simulink model "SPGF_FSK_0000_R2020b"  (R2020b)
settings: Solver=ode4  StartTime=0.0  StopTime=1.4  FixedStep=50e-6/50  RelTol=1e-3  EnableMultiTasking=on
undefined symbols (not defined in the file): D11, Delta
libraries: powerlib x2546, powerlib_meascontrol x183, simulink x24
(part 1 of 34)
settings Model: SimulationMode=accelerator  Creator=Anastasia  LastModifiedBy=Fedot
settings DataIOCC: SaveFormat=Array  SaveOutput=off  SignalLogging=off  DSMLogging=off  SaveTime=off  ReturnWorkspaceOutputs=off
settings OptimizationCC: BlockReduction=off  OptimizeBlockIOStorage=off  BufferReuse=off  GlobalBufferReuse=off  ExpressionFolding=off  LocalBlockOutputs=off  EfficientMapNaN2IntZero=off  LifeSpan=inf
settings DebuggingCC: UnderspecifiedInitializationDetection=Classic  MergeDetectMultiDrivingBlocksExec=none  SolverPrmCheckMsg=warning  UnconnectedInputMsg=none  UnconnectedOutputMsg=none  UnconnectedLineMsg=none  AllowSymbolicDim=off  StateNameClashWarn=warning  SFUnexpectedBacktrackingDiag=warning  SFNoUnconditionalDefaultTransitionDiag=warning  SFExecutionAtInitializationDiag=none  ArithmeticOperatorsInVariantConditions=warning
settings HardwareCC: ProdBitPerPointer=32  ProdBitPerSizeT=32  ProdBitPerPtrDiffT=32  ProdLargestAtomicFloat=None  ProdIntDivRoundTo=Undefined  ProdEndianess=Unspecified  ProdWordSize=32  ProdHWDeviceType=32-bit Generic  TargetBitPerPointer=64  TargetBitPerSizeT=64  TargetBitPerPtrDiffT=64  TargetLongLongMode=on  TargetIntDivRoundTo=Zero  TargetEndianess=LittleEndian  TargetWordSize=64  TargetHWDeviceType=MATLAB Host  ProdEqTarget=off
settings ModelReferenceCC: PropagateSignalLabelsOutOfModel=off
settings SFSimCC: SimUseLocalCustomCode=off  CustomCodeUndefinedFunction=UseInterfaceOnly
settings RTWCC: RTWUseLocalCustomCode=off
settings CodeAppCC: MaxIdLength=128  StateflowObjectComments=on
settings GRTTargetCC: TargetLangStandard=C89/C90 (ANSI)  CombineOutputUpdateFcns=off  GRTInterface=on
settings ConfigComp: CovMetricSettings=dw  CovSaveCumulativeToWorkspaceVar=on  CovSaveSingleToWorkspaceVar=on  CovExternalEMLEnable=off
settings SimscapeCC: SimscapeNormalizeSystem=off

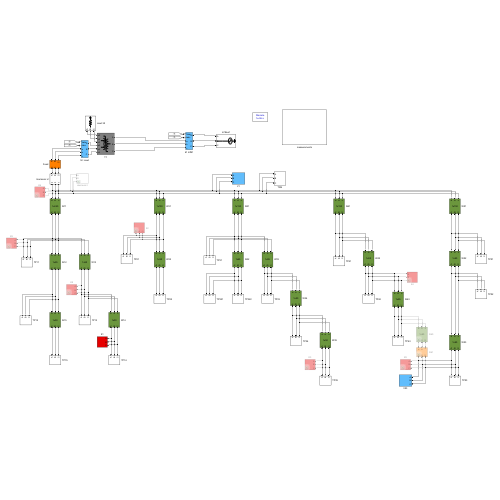
[thumbnail: Simulink's stored preview of the top-level diagram]
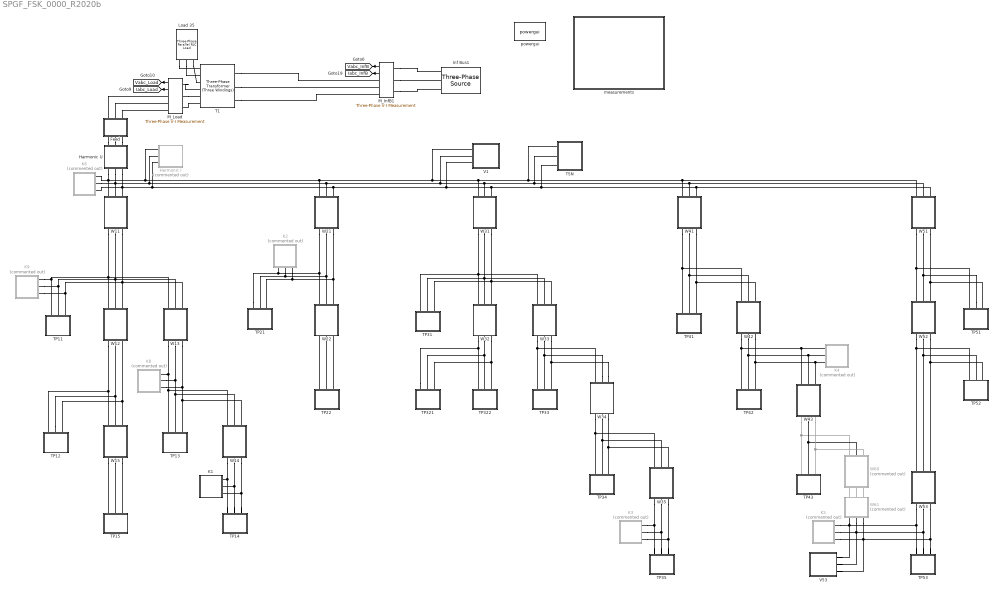
== system SPGF_FSK_0000_R2020b ==
  Feed : Subsystem
      mask Display:
      | port_label('lconn',1,'A');
      | port_label('lconn',2,'B');
      | port_label('lconn',3,'C');
      | 
      | port_label('rconn',1,'a');
      | port_label('rconn',2,'b');
      | port_label('rconn',3,'c');
  Harmonic I : Subsystem  Commented=on  mask(Three-Phase Harmonic Current Source){ActiveABC=[1 0 0], Frequency=50, PhaseABC=[0 -120 120], HN=[5, 7, 11, 13, 17], Current=19.26, Percent=[2.84, 2.42, 1.67, 0.74, 0.3], PhaseH=[0 0 0 0 0]}
      mask prompts: ActiveABC "Active phase of source [A, B, C]"; Frequency "Frequency f [Hz] :"; PhaseABC "Current phase [phA, phB, phC] [degree]"; HN "Vector of harmonic numbers [5, 7, 11, 13 ...] :"; Current "Base current rms [A] :"; Percent "Percent of harmanic in base current [%] :"; PhaseH "Phase of harmonic current [degree] :"
      mask help: Add harmonic to current
      mask init:
      | ActiveA = ActiveABC(1);
      |     ActiveB = ActiveABC(2);
      |     ActiveC = ActiveABC(3);
      |     PhaseA = PhaseABC(1);
      |     PhaseB = PhaseABC(2);
      |     PhaseC = PhaseABC(3);
  Harmonic U : Subsystem  mask(Three-Phase Harmonic Voltage Source){EnableH=off, ActiveABC=[1, 1, 1], Frequency=50, PhaseABC=[0 -120 120], HN=[5, 7, 11, 13, 17], Voltage=1000, Percent=[2.84, 2.42, 1.67, 0.74, 0.3].*1.5, PhaseH=[0 0 0 0 0]}
      mask prompts: EnableH "Enable harmonic voltage source"; ActiveABC "Active phase of source [A, B, C]"; Frequency "Frequency f [Hz] :"; PhaseABC "Voltage phase [phA, phB, phC] [degree]"; HN "Vector of harmonic numbers [5, 7, 11, 13 ...] :"; Voltage "Base Voltage rms [V] :"; Percent "Percent of harmanic in base voltage [%] :"; PhaseH "Phase of harmonic voltage [degree] :"
      mask help:
      | The block allows to add harmonic signals to voltage.
      | The block is connected in series.
      mask init:
      | PhaseA = PhaseABC(1);
      |     PhaseB = PhaseABC(2);
      |     PhaseC = PhaseABC(3);
      |     ActiveA = ActiveABC(1);
      |     ActiveB = ActiveABC(2);
      |     ActiveC = ActiveABC(3);
      mask Callback EnableH:
      | base_block_name = gcb;
      |     enable = get_param(base_block_name, 'EnableH');
      |     if strcmp(enable, 'on')
      |         set_param([base_block_name, '/harmonic'],'Commented','off');
      |         set_param([base_block_name, '/shunt'],'Commented','on');
      |     else
      |         set_param([base_block_name, '/harmonic'],'Commented','on');
      |         set_param([base_block_name, '/shunt'],'Commented','off');
      |     end
  Inf Bus1 : powerlib/Electrical Sources/Three-Phase Source  InternalConnection=Yg  VoltagePhases=off  Voltage=(115500)*1  PhaseAngle=0  Voltage_phases=[25e3 25e3 25e3]/sqrt(3)  PhaseAngles_phases=[0 -120 +120]  Frequency=50  NonIdealSource=on  SpecifyImpedance=off  Resistance=0  Inductance=0  ShortCircuitLevel=100e6  BaseVoltage=115.5e3  XRratio=7  BusType=swing  Pref=0  Qref=0  Prefabc=[10e3, 10e3, 10e3]  Qrefabc=[0, 0, 0]  Qmin=-inf  Qmax=inf
  K1 : Subsystem
  K2 : Subsystem  Commented=on
  K3 : Subsystem  Commented=on
  K4 : Subsystem  Commented=on
  K5 : Subsystem  Commented=on
  K6 : Subsystem  Commented=on
  K8 : Subsystem  Commented=on
  K9 : Subsystem  Commented=on
  Load 35 : powerlib/Elements/Three-Phase Parallel RLC Load  LConnTagsString=A|B|C  Configuration=Y (grounded)  NominalVoltage=(38435.4)*1  Vabc=[1e3 1e3 1e3]  Vabcp=[1e3 1e3 1e3]  NominalFrequency=50  UnbalancedPower=off  ActivePower=1e6  InductivePower=0  CapacitivePower=0  Pabc=[10e3 9e3 11e3]  QLabc=[100 90 110]  QCabc=[100 90 110]  Pabcp=[10e3 9e3 11e3]  QLabcp=[100 90 110]  QCabcp=[100 90 110]  Measurements=None  LoadType=constant PQ
  M_InfB1 : powerlib/Measurements/Three-Phase V-I Measurement  VoltageMeasurement=phase-to-ground  SetLabelV=off  LabelV=Vabc  Vpu=off  VpuLL=off  CurrentMeasurement=yes  SetLabelI=off  LabelI=Iabc  Ipu=off  Pbase=100e6  Vbase=500e3  OutputType=Complex  PhasorSimulation=off  PSBequivalent=0
  M_Load : powerlib/Measurements/Three-Phase V-I Measurement  VoltageMeasurement=phase-to-ground  SetLabelV=off  LabelV=Vabc  Vpu=off  VpuLL=off  CurrentMeasurement=yes  SetLabelI=off  LabelI=Iabc  Ipu=off  Pbase=100e6  Vbase=500e3  OutputType=Complex  PhasorSimulation=off  PSBequivalent=0
  T1 : powerlib/Elements/Three-Phase Transformer (Three Windings)  Winding1Connection=Yg  Winding2Connection=Y  Winding3Connection=Delta (D11)  CoreType=Three single-phase transformers  SetSaturation=on  Hysteresis=off  DataFile='hysteresis'  SetInitialFlux=off  Measurements=None  UNITS=pu  NominalPower=[20e6 , 50 ]  Winding1=[115.5e3 , 0.003175 , 0.01025 ]  Winding2=[ 38.5e3 , 0.003175 , -0.0025]  Winding3="[ 11e3 , 0.003175 ,  0.0125 ]"  Rm=444.444  Lm=40  L0=2  Saturation=[0 0;0.01774 0.324129;0.0487637 0.61284;0.0980856 0.825118;0.2 1;0.309543 1.08024;0.652348 1.17344;2.0357 1.26115;6.0215 1.36094;12.4388 1.49469]  InitialFluxes=[-0.996027177222096 0.502063669050077 0.493963508171988]  BreakLoop=on  DiscreteSolver=Trapezoidal iterative  DataType=off  TransfoNumber=1
  TP11 : Subsystem
  TP12 : Subsystem
  TP13 : Subsystem
  TP14 : Subsystem
  TP15 : Subsystem
  TP21 : Subsystem
  TP22 : Subsystem
  TP31 : Subsystem
  TP321 : Subsystem
  TP322 : Subsystem
  TP33 : Subsystem
  TP34 : Subsystem
  TP35 : Subsystem
  TP41 : Subsystem
  TP42 : Subsystem
  TP43 : Subsystem
  TP51 : Subsystem
  TP52 : Subsystem
  TP53 : Subsystem
  TSN : Subsystem
  V1 : Subsystem
  V53 : Subsystem
  W11 : Subsystem
      mask Display:
      | port_label('lconn',1,'A');
      | port_label('lconn',2,'B');
      | port_label('lconn',3,'C');
      | 
      | port_label('rconn',1,'a');
      | port_label('rconn',2,'b');
      | port_label('rconn',3,'c');
      | disp('1x240');
  W12 : Subsystem
      mask Display:
      | port_label('lconn',1,'A');
      | port_label('lconn',2,'B');
      | port_label('lconn',3,'C');
      | 
      | port_label('rconn',1,'a');
      | port_label('rconn',2,'b');
      | port_label('rconn',3,'c');
      | disp('1x95');
  W13 : Subsystem
      mask Display:
      | port_label('lconn',1,'A');
      | port_label('lconn',2,'B');
      | port_label('lconn',3,'C');
      | 
      | port_label('rconn',1,'a');
      | port_label('rconn',2,'b');
      | port_label('rconn',3,'c');
      | disp('1x95');
  W14 : Subsystem
      mask Display:
      | port_label('lconn',1,'A');
      | port_label('lconn',2,'B');
      | port_label('lconn',3,'C');
      | 
      | port_label('rconn',1,'a');
      | port_label('rconn',2,'b');
      | port_label('rconn',3,'c');
      | disp('1x50');
  W15 : Subsystem
      mask Display:
      | port_label('lconn',1,'A');
      | port_label('lconn',2,'B');
      | port_label('lconn',3,'C');
      | 
      | port_label('rconn',1,'a');
      | port_label('rconn',2,'b');
      | port_label('rconn',3,'c');
      | disp('1x50');
  W21 : Subsystem
      mask Display:
      | port_label('lconn',1,'A');
      | port_label('lconn',2,'B');
      | port_label('lconn',3,'C');
      | 
      | port_label('rconn',1,'a');
      | port_label('rconn',2,'b');
      | port_label('rconn',3,'c');
      | disp('1x150');
  W22 : Subsystem
      mask Display:
      | port_label('lconn',1,'A');
      | port_label('lconn',2,'B');
      | port_label('lconn',3,'C');
      | 
      | port_label('rconn',1,'a');
      | port_label('rconn',2,'b');
      | port_label('rconn',3,'c');
      | disp('1x95');
  W31 : Subsystem
      mask Display:
      | port_label('lconn',1,'A');
      | port_label('lconn',2,'B');
      | port_label('lconn',3,'C');
      | 
      | port_label('rconn',1,'a');
      | port_label('rconn',2,'b');
      | port_label('rconn',3,'c');
      | disp('1x150');
  W32 : Subsystem
      mask Display:
      | port_label('lconn',1,'A');
      | port_label('lconn',2,'B');
      | port_label('lconn',3,'C');
      | 
      | port_label('rconn',1,'a');
      | port_label('rconn',2,'b');
      | port_label('rconn',3,'c');
      | disp('1x95');
  W33 : Subsystem
      mask Display:
      | port_label('lconn',1,'A');
      | port_label('lconn',2,'B');
      | port_label('lconn',3,'C');
      | 
      | port_label('rconn',1,'a');
      | port_label('rconn',2,'b');
      | port_label('rconn',3,'c');
      | disp('1x95');
  W34 : Subsystem
      mask Display:
      | port_label('lconn',1,'A');
      | port_label('lconn',2,'B');
      | port_label('lconn',3,'C');
      | 
      | port_label('rconn',1,'a');
      | port_label('rconn',2,'b');
      | port_label('rconn',3,'c');
      | disp('1x50');
  W35 : Subsystem
      mask Display:
      | port_label('lconn',1,'A');
      | port_label('lconn',2,'B');
      | port_label('lconn',3,'C');
      | 
      | port_label('rconn',1,'a');
      | port_label('rconn',2,'b');
      | port_label('rconn',3,'c');
      | disp('1x50');
  W41 : Subsystem
      mask Display:
      | port_label('lconn',1,'A');
      | port_label('lconn',2,'B');
      | port_label('lconn',3,'C');
      | 
      | port_label('rconn',1,'a');
      | port_label('rconn',2,'b');
      | port_label('rconn',3,'c');
      | disp('1x150');
  W42 : Subsystem
      mask Display:
      | port_label('lconn',1,'A');
      | port_label('lconn',2,'B');
      | port_label('lconn',3,'C');
      | 
      | port_label('rconn',1,'a');
      | port_label('rconn',2,'b');
      | port_label('rconn',3,'c');
      | disp('1x95');
  W43 : Subsystem
      mask Display:
      | port_label('lconn',1,'A');
      | port_label('lconn',2,'B');
      | port_label('lconn',3,'C');
      | 
      | port_label('rconn',1,'a');
      | port_label('rconn',2,'b');
      | port_label('rconn',3,'c');
      | disp('1x95');
  W51 : Subsystem
      mask Display:
      | port_label('lconn',1,'A');
      | port_label('lconn',2,'B');
      | port_label('lconn',3,'C');
      | 
      | port_label('rconn',1,'a');
      | port_label('rconn',2,'b');
      | port_label('rconn',3,'c');
      | disp('1x150');
  W52 : Subsystem
      mask Display:
      | port_label('lconn',1,'A');
      | port_label('lconn',2,'B');
      | port_label('lconn',3,'C');
      | 
      | port_label('rconn',1,'a');
      | port_label('rconn',2,'b');
      | port_label('rconn',3,'c');
      | disp('1x95');
  W53 : Subsystem
      mask Display:
      | port_label('lconn',1,'A');
      | port_label('lconn',2,'B');
      | port_label('lconn',3,'C');
      | 
      | port_label('rconn',1,'a');
      | port_label('rconn',2,'b');
      | port_label('rconn',3,'c');
      | disp('1x95');
  W60 : Subsystem  Commented=on
      mask Display:
      | port_label('lconn',1,'A');
      | port_label('lconn',2,'B');
      | port_label('lconn',3,'C');
      | 
      | port_label('rconn',1,'a');
      | port_label('rconn',2,'b');
      | port_label('rconn',3,'c');
      | disp('1x95');
  W61 : Subsystem  Commented=on
      mask Display:
      | port_label('lconn',1,'A');
      | port_label('lconn',2,'B');
      | port_label('lconn',3,'C');
      | 
      | port_label('rconn',1,'a');
      | port_label('rconn',2,'b');
      | port_label('rconn',3,'c');
  measurements : Subsystem  mask{FTime=0.02/40}
      mask prompts: FTime "Fourier Sample Time"
  powergui : powerlib/powergui  Priority=1  SimulationMode=Discrete  SampleTime=50e-6/50  frequency=60  Iterations=100  frequencyindice=0  Pbase=1e+06  ErrMax=0.0001  UnitsV=kV  UnitsW=MW  buscounter=0  FunctionMessages=off  echomessages=off  EnableUseOfTLC=off  CurrentSourceSwitches=off  DisableSnubberDevices=off  DisableRonSwitches=off  DisableVfSwitches=off  DisplayEquations=off  AutomaticDiscreteSolvers=off  SolverType=Backward Euler  Interpol=off  ExternalGateDelay=off  methode=off  Ts=0  x0status=blocks  SPID=off  SwTol=0  HookPort=off  NonlinearTolerance=1e-4  nMaxIteration=100  ContinueOnMaxIteration=off  RestoreLinks=warning  ResistiveCurrentMeasurement=off  Frange=[0:2:500]  Ylog=off  Xlog=on  ShowGrid=off  save=off  variable=ZData  structure=0  ZoomFFT=off  StartTime=0.0  cycles=1  DisplayStyle=1  fundamental=60  FreqAxis=off  MaxFrequency=1000  frequencyindicesteady=1  RmsSteady=2  display=off
  tag scope: Iabc_InfB=global, Iabc_Load=global, Vabc_InfB=global, Vabc_Load=global
  wires:
  M_InfB1/1 -> [Vabc_InfB]
  M_InfB1/2 -> [Iabc_InfB]
  M_Load/1 -> [Vabc_Load]
  M_Load/2 -> [Iabc_Load]
  connections:
  M_InfB1/LConn1 -- Inf Bus1/RConn1
  TP12/RConn2 -- W15/RConn2 -- W12/LConn2
  W12/LConn3 -- W15/RConn3 -- TP12/RConn3
  W15/RConn1 -- TP12/RConn1 -- W12/LConn1
  W13/LConn1 -- K8/LConn1 -- W14/RConn1 -- TP13/RConn1
  W13/LConn2 -- K8/LConn2 -- W14/RConn2 -- TP13/RConn2
  W14/RConn3 -- K8/LConn3 -- W13/LConn3 -- TP13/RConn3
  W14/LConn1 -- TP14/RConn1 -- K1/LConn1
  K1/LConn2 -- TP14/RConn2 -- W14/LConn2
  TP21/RConn1 -- K2/LConn1 -- W22/RConn1 -- W21/LConn1
  TP21/RConn3 -- K2/LConn3 -- W22/RConn3 -- W21/LConn3
  TP21/RConn2 -- K2/LConn2 -- W22/RConn2 -- W21/LConn2
  W33/RConn2 -- TP31/RConn2 -- W32/RConn2 -- W31/LConn2
  W33/RConn3 -- TP31/RConn3 -- W32/RConn3 -- W31/LConn3
  W33/RConn1 -- TP31/RConn1 -- W32/RConn1 -- W31/LConn1
  TP321/RConn1 -- TP322/RConn1 -- W32/LConn1
  TP321/RConn2 -- TP322/RConn2 -- W32/LConn2
  TP322/RConn3 -- TP321/RConn3 -- W32/LConn3
  W34/RConn3 -- TP33/RConn3 -- W33/LConn3
  W34/RConn1 -- TP33/RConn1 -- W33/LConn1
  W34/RConn2 -- TP33/RConn2 -- W33/LConn2
  W35/RConn3 -- TP34/RConn3 -- W34/LConn3
  W35/RConn1 -- TP34/RConn1 -- W34/LConn1
  W35/RConn2 -- TP34/RConn2 -- W34/LConn2
  TP35/RConn3 -- K3/LConn3 -- W35/LConn3
  TP35/RConn1 -- K3/LConn1 -- W35/LConn1
  TP35/RConn2 -- K3/LConn2 -- W35/LConn2
  W42/RConn2 -- TP41/RConn2 -- W41/LConn2
  W42/RConn1 -- TP41/RConn1 -- W41/LConn1
  W42/RConn3 -- TP41/RConn3 -- W41/LConn3
  W43/RConn3 -- K4/LConn3 -- TP42/RConn3 -- W42/LConn3
  W43/RConn1 -- K4/LConn1 -- TP42/RConn1 -- W42/LConn1
  TP42/RConn2 -- W42/LConn2 -- K4/LConn2 -- W43/RConn2
  W60/RConn1 -- TP43/RConn1 -- W43/LConn1
  TP43/RConn2 -- W60/RConn2 -- W43/LConn2
  W60/RConn3 -- TP43/RConn3 -- W43/LConn3
  W51/LConn3 -- TP51/RConn3 -- W52/RConn3
  W52/RConn1 -- TP51/RConn1 -- W51/LConn1
  TP51/RConn2 -- W51/LConn2 -- W52/RConn2
  TP52/RConn2 -- W53/RConn2 -- W52/LConn2
  TP52/RConn3 -- W53/RConn3 -- W52/LConn3
  TP52/RConn1 -- W53/RConn1 -- W52/LConn1
  T1/LConn2 -- M_InfB1/RConn2
  M_InfB1/LConn2 -- Inf Bus1/RConn2
  Load 35/LConn2 -- T1/RConn2
  M_InfB1/LConn3 -- Inf Bus1/RConn3
  T1/LConn3 -- M_InfB1/RConn3
  T1/LConn1 -- M_InfB1/RConn1
  Load 35/LConn1 -- T1/RConn1
  Load 35/LConn3 -- T1/RConn3
  W15/LConn1 -- TP15/RConn1
  W15/LConn2 -- TP15/RConn2
  TP22/RConn3 -- W22/LConn3
  TP22/RConn1 -- W22/LConn1
  TP22/RConn2 -- W22/LConn2
  W15/LConn3 -- TP15/RConn3
  M_Load/LConn3 -- T1/RConn6
  M_Load/LConn2 -- T1/RConn5
  M_Load/LConn1 -- T1/RConn4
  Feed/LConn1 -- M_Load/RConn1
  Feed/LConn2 -- M_Load/RConn2
  Feed/LConn3 -- M_Load/RConn3
  W14/LConn3 -- TP14/RConn3 -- K1/LConn3
  W11/LConn3 -- K9/LConn3 -- TP11/RConn3 -- W13/RConn3 -- W12/RConn3
  W11/LConn1 -- K9/LConn1 -- TP11/RConn1 -- W13/RConn1 -- W12/RConn1
  W61/LConn2 -- K5/LConn2 -- V53/LConn2 -- TP53/RConn2 -- W53/LConn2
  W61/LConn1 -- K5/LConn1 -- V53/LConn1 -- TP53/RConn1 -- W53/LConn1
  W61/LConn3 -- K5/LConn3 -- V53/LConn3 -- TP53/RConn3 -- W53/LConn3
  Harmonic U/RConn1 -- K6/LConn1 -- W11/RConn1 -- Harmonic I/LConn1 -- W21/RConn1 -- V1/LConn1 -- W31/RConn1 -- TSN/LConn1 -- W51/RConn1 -- W41/RConn1
  Harmonic I/LConn2 -- Harmonic U/RConn2 -- K6/LConn2 -- W11/RConn2 -- W21/RConn2 -- V1/LConn2 -- W51/RConn2 -- W41/RConn2 -- TSN/LConn2 -- W31/RConn2
  TSN/LConn3 -- Harmonic I/LConn3 -- Harmonic U/RConn3 -- W11/RConn3 -- K6/LConn3 -- W21/RConn3 -- V1/LConn3 -- W31/RConn3 -- W51/RConn3 -- W41/RConn3
  W61/RConn1 -- W60/LConn1
  W61/RConn2 -- W60/LConn2
  W61/RConn3 -- W60/LConn3
  TP11/RConn2 -- K9/LConn2 -- W11/LConn2 -- W12/RConn2 -- W13/RConn2
  Feed/RConn1 -- Harmonic U/LConn1
  Feed/RConn2 -- Harmonic U/LConn2
  Feed/RConn3 -- Harmonic U/LConn3

== system SPGF_FSK_0000_R2020b/Feed ==
  Q : Subsystem
  A : PMIOPort  Side=Left
  B : PMIOPort  Port=2  Side=Left
  C : PMIOPort  Port=3  Side=Left
  a : PMIOPort  Port=4  Side=Right
  b : PMIOPort  Port=5  Side=Right
  c : PMIOPort  Port=6  Side=Right
  connections:
  Q/RConn3 -- C/RConn1
  Q/RConn2 -- B/RConn1
  Q/LConn2 -- b/RConn1
  Q/LConn1 -- a/RConn1
  Q/LConn3 -- c/RConn1
  Q/RConn1 -- A/RConn1

== system SPGF_FSK_0000_R2020b/Harmonic I ==
  Clock : Clock
  Constant1 : Constant  Value=PhaseB
  Constant2 : Constant  Value=PhaseC
  Constant3 : Constant  Value=PhaseA
  Constant4 : Constant  Value=ActiveA
  Constant5 : Constant  Value=ActiveB
  Constant6 : Constant  Value=ActiveC
  Ground : powerlib/Elements/Ground  LConnTagsString=a
  In A : powerlib/Electrical Sources/Controlled Current Source  Initialize=on  Source_Type=AC  Amplitude=0  Phase=0  Frequency=50  Measurements=None
  In B : powerlib/Electrical Sources/Controlled Current Source  Initialize=on  Source_Type=AC  Amplitude=0  Phase=-120  Frequency=50  Measurements=None
  In C : powerlib/Electrical Sources/Controlled Current Source  Initialize=on  Source_Type=AC  Amplitude=0  Phase=120  Frequency=50  Measurements=None
  Product1 : Product
  Product15 : Product
  Product2 : Product
  R : powerlib/Elements/Three-Phase Series RLC Branch  LConnTagsString=A|B|C  RConnTagsString=A|B|C  BranchType=R  Resistance=1e6  Inductance=0  Capacitance=0  Measurements=None
  Subsystem1 : Subsystem
  Subsystem2 : Subsystem
  Subsystem3 : Subsystem
  Sum of Elements : Sum  Inputs=+
  Sum of Elements1 : Sum  Inputs=+
  Sum of Elements2 : Sum  Inputs=+
  A : PMIOPort  Tag=PMCPort  Side=Left
  B : PMIOPort  Tag=PMCPort  Port=2  Side=Left
  C : PMIOPort  Tag=PMCPort  Port=3  Side=Left
  wires:
  Product2/1 -> In C/1
  Constant6/1 -> Product2/1
  Product1/1 -> In B/1
  Constant5/1 -> Product1/1
  Product15/1 -> In A/1
  Constant4/1 -> Product15/1
  Subsystem3/1(o) -> Sum of Elements/1
  Subsystem1/1(o) -> Sum of Elements1/1
  Subsystem2/1(o) -> Sum of Elements2/1
  Sum of Elements/1 -> Product15/2
  Sum of Elements1/1 -> Product1/2
  Sum of Elements2/1 -> Product2/2
  Constant3/1 -> Subsystem3/2(phase)
  Constant1/1 -> Subsystem1/2(phase)
  Clock/1 -> Subsystem3/1(clock), Subsystem2/1(clock), Subsystem1/1(clock)
  Constant2/1 -> Subsystem2/2(phase)
  connections:
  R/RConn1 -- In A/RConn1
  In B/RConn1 -- R/RConn2
  R/RConn3 -- In C/RConn1
  In C/LConn1 -- Ground/LConn1 -- In A/LConn1 -- In B/LConn1
  B/RConn1 -- R/LConn2
  C/RConn1 -- R/LConn3
  A/RConn1 -- R/LConn1

== system SPGF_FSK_0000_R2020b/Harmonic U ==
  harmonic : Subsystem  Commented=on
  shunt : Subsystem
  A : PMIOPort  Tag=PMCPort  Side=Left
  B : PMIOPort  Tag=PMCPort  Port=2  Side=Left
  C : PMIOPort  Tag=PMCPort  Port=3  Side=Left
  a : PMIOPort  Port=4  Side=Right
  b : PMIOPort  Port=5  Side=Right
  c : PMIOPort  Port=6  Side=Right
  connections:
  harmonic/LConn1 -- shunt/LConn3 -- A/RConn1
  harmonic/RConn3 -- shunt/RConn3 -- c/RConn1
  b/RConn1 -- harmonic/RConn2 -- shunt/RConn2
  a/RConn1 -- harmonic/RConn1 -- shunt/RConn1
  harmonic/LConn3 -- shunt/LConn2 -- C/RConn1
  harmonic/LConn2 -- shunt/LConn1 -- B/RConn1

== system SPGF_FSK_0000_R2020b/K1 ==
  fault : Subsystem  mask{FaultA=on, FaultB=off, FaultC=off, FaultResistance=0.0001, GroundResistance=1e-03, SnubberResistance=1e6, SnubberCapacitance=inf, TransitionTimes=[0.2 0.8], TheoryOfArc=Peters & Slepian, ArcingVoltage=6000, TypeOfPause=None, NoiseSampleTime=0.04, NoiseSeed=23345, PulsePeriod=0.2, PulseWidth=20, PhaseDelay=0.2, SwitchTimes=[0.2 0.225 0.5 0.6], LimitArcNum=off, ArcingNumber=2, AddTimeDelay=off, TimeDelay=[0 0.1 0.2 ]}
      mask prompts: FaultA "Phase A Fault"; FaultB "Phase B Fault"; FaultC "Phase C Fault"; FaultResistance "Fault resistance Ron (ohms) :"; GroundResistance "Ground resistance Rg (ohms) :"; SnubberResistance "Snubbers resistance Rp (ohms) :"; SnubberCapacitance "Snubbers capacitance Cp (F) :"; TransitionTimes "Transition times (s) :"; TheoryOfArc "Theory of the arcing ground"; ArcingVoltage "Voltage of the arcing (V) :"; TypeOfPause "Add pause in the arcing ground"; NoiseSampleTime "Sample time of white noise (s) :"; NoiseSeed "Seed of white noise"; PulsePeriod "Period of pulses (s) :"; PulseWidth "Width of pulse (% of period) :"; PhaseDelay "Phase delay (sec) :"; SwitchTimes "Switch times (sec) [1,0,1,0...] :"; LimitArcNum "Limit number of arcing [N] :"; ArcingNumber "Number of uprising arcing"; AddTimeDelay "Add time delay :"; TimeDelay "Time delay between arc (sec) [1xN] :"
      mask init:
      | FaultA = double(FaultA);
      | FaultB = double(FaultB);
      | FaultC = double(FaultC);
      | if (FaultA == 1)
      |     FaultPhase = 1;
      | elseif (FaultB == 1)
      |     FaultPhase = 2;    
      | elseif (FaultC == 1)
      |     FaultPhase = 3; 
      | else
      |     FaultPhase = 4; 
      | end
      |     BeginFaultTime = TransitionTimes(1);
      |     EndFaultTime = TransitionTimes(2);
      | if (length(ArcingVoltage) == 1)
      |     Slope = 0;
      | end
      | if (length(ArcingVoltage) > 1)
      |     Slope = (ArcingVoltage(2)-ArcingVoltage(1))/(EndFaultTime-BeginFaultTime);
      | end
      | 
      | SwitchStatus(1) = 0;
      | for i=1:length(SwitchTimes)
      |     SwitchStatus(i+1) = double(~(logical(SwitchStatus(i))));
      | end
      | SwitchTimes = [0,SwitchTimes];
      | 
      | LimitArcNum = double(LimitArcNum);
      | AddTimeDelay = double(AddTimeDelay);
      | 
      | if (AddTimeDelay == 0)
      |     TimeDelay = zeros(1,ArcingNumber);
      | end
      settings: CloseFcn=|
      | en = get_param(gcb,'MaskEnables');
      | set_param(gcb,'MaskEnables',en)
      | clear enab en;
      settings: MoveFcn=|
      | en = get_param(gcb,'MaskEnables');
      | set_param(gcb,'MaskEnables',en)
      | clear enab en;
      mask Callback FaultA:
      | enab = get_param(gcb,'FaultA');
      | en = get_param(gcb,'MaskEnables');
      | % Set the 'MaskVisililities' property for each parameters
      | if strcmp(enab,'on')
      |     en{2}='off';
      |     en{3}='off';
      | % set_param(gcb,'MaskVisibilities',{'on','on','on','on','on','on','on','on','on','off','on','',''});
      | else
      |     en{2}='on';
      |     en{3}='on';
      | % set_param(gcb,'MaskVisibilities',{'on','on','on','on','on','on','on','on','on','on','on','',''});
      | end
      | set_param(gcb,'MaskEnables',en)
      | clear enab en;
      mask Callback FaultB:
      | enab = get_param(gcb,'FaultB');
      | en = get_param(gcb,'MaskEnables');
      | % Set the 'MaskVisililities' property for each parameters
      | if strcmp(enab,'on')
      |     en{1}='off';
      |     en{3}='off';
      | % set_param(gcb,'MaskVisibilities',{'on','on','on','on','on','on','on','on','on','off','on','',''});
      | else
      |     en{1}='on';
      |     en{3}='on';
      | % set_param(gcb,'MaskVisibilities',{'on','on','on','on','on','on','on','on','on','on','on','',''});
      | end
      | set_param(gcb,'MaskEnables',en)
      | clear enab en;
      mask Callback FaultC:
      | enab = get_param(gcb,'FaultC');
      | en = get_param(gcb,'MaskEnables');
      | % Set the 'MaskVisililities' property for each parameters
      | if strcmp(enab,'on')
      |     en{1}='off';
      |     en{2}='off';
      | % set_param(gcb,'MaskVisibilities',{'on','on','on','on','on','on','on','on','on','off','on','',''});
      | else
      |     en{1}='on';
      |     en{2}='on';
      | % set_param(gcb,'MaskVisibilities',{'on','on','on','on','on','on','on','on','on','on','on','',''});
      | end
      | set_param(gcb,'MaskEnables',en)
      | clear enab en;
      mask TypeOptions TheoryOfArc: None | Petersen | Peters & Slepian
      mask Callback TheoryOfArc:
      | enab = get_param(gcb,'TheoryOfArc');
      | en = get_param(gcb,'MaskEnables');
      | % Set the 'MaskVisililities' property for each parameters
      | if strcmp(enab,'None')
      |     en{10}='off';
      | % set_param(gcb,'MaskVisibilities',{'on','on','on','on','on','on','on','on','on','off','on','',''});
      | else
      |     en{10}='on';
      | % set_param(gcb,'MaskVisibilities',{'on','on','on','on','on','on','on','on','on','on','on','',''});
      | end
      | set_param(gcb,'MaskEnables',en)
      | clear enab en;
      mask TypeOptions TypeOfPause: None | White Noise | Pulse Generator | Time Dependent Pulses
      mask Callback TypeOfPause:
      | enab = get_param(gcb,'TypeOfPause');
      | en = get_param(gcb,'MaskVisibilities');
      | % Set the 'MaskVisibilities' property for each parameters
      | if strcmp(enab,'None')
      |     en{12} = 'off';
      |     en{13} = 'off';
      |     en{14} = 'off';
      |     en{15} = 'off';
      |     en{16} = 'off';
      |     en{17} = 'off';
      | % set_param(gcb,'MaskEnables',{'on','on','on','on','on','on','on','on','on','on','on','on','on'});
      | elseif strcmp(enab,'White Noise')
      |     en{12} = 'on';
      |     en{13} = 'on';
      |     en{14} = 'off';
      |     en{15} = 'off';
      |     en{16} = 'off';
      |     en{17} = 'off';
      | elseif strcmp(enab,'Pulse Generator')
      |     en{12} = 'off';
      |     en{13} = 'off';
      |     en{14} = 'on';
      |     en{15} = 'on';
      |     en{16} = 'on';
      |     en{17} = 'off';
      | else
      |     en{12} = 'off';
      |     en{13} = 'off';
      |     en{14} = 'off';
      |     en{15} = 'off';
      |     en{16} = 'off';
      |     en{17} = 'on';
      | % set_param(gcb,'Maskenables',{'on','on','on','on','on','on','on','on','on','on','on','off','off'});
      | end
      | set_param(gcb,'MaskVisibilities',en);
      | clear enab en;
      mask Callback LimitArcNum:
      | enab = get_param(gcb,'LimitArcNum');
      | en = get_param(gcb,'MaskVisibilities');
      | % Set the 'MaskVisibilities' property for each parameters
      | if strcmp(enab,'on')
      |     en{19} = 'on';
      |     en{20} = 'on';
      |     en{21} = 'on';
      | else
      |     en{19} = 'off';
      |     en{20} = 'off';
      |     set_param(gcb,'AddTimeDelay','off');
      |     en{21} = 'off';
      | % set_param(gcb,'Maskenables',{'on','on','on','on','on','on','on','on','on','on','on','off','off'});
      | end
      | set_param(gcb,'MaskVisibilities',en);
      | clear enab en;
      mask Callback AddTimeDelay:
      | enab = get_param(gcb,'AddTimeDelay');
      | en = get_param(gcb,'MaskVisibilities');
      | % Set the 'MaskVisibilities' property for each parameters
      | if strcmp(enab,'on')
      |     en{21} = 'on';
      | else
      |     en{21} = 'off';
      | % set_param(gcb,'Maskenables',{'on','on','on','on','on','on','on','on','on','on','on','off','off'});
      | end
      | set_param(gcb,'MaskVisibilities',en);
      | clear enab en;
      mask Display:
      | % port_label('input',1,'Iabc');
      | 
      | port_label('lconn',1,'A');
      | port_label('lconn',2,'B');
      | port_label('lconn',3,'C');
      | 
      | disp('   ПДЗ    ');
  meas : Subsystem
  A : PMIOPort  Side=Left
  B : PMIOPort  Port=2  Side=Left
  C : PMIOPort  Port=3  Side=Left
  connections:
  meas/LConn3 -- C/RConn1
  meas/LConn1 -- A/RConn1
  meas/LConn2 -- B/RConn1
  fault/LConn3 -- meas/RConn3
  fault/LConn2 -- meas/RConn2
  fault/LConn1 -- meas/RConn1

== system SPGF_FSK_0000_R2020b/K2 ==
  fault : Subsystem  mask{FaultA=on, FaultB=off, FaultC=off, FaultResistance=0.0001, GroundResistance=1e-03, SnubberResistance=1e6, SnubberCapacitance=inf, TransitionTimes=[0.2 0.8], TheoryOfArc=None, ArcingVoltage=6000, TypeOfPause=None, NoiseSampleTime=0.04, NoiseSeed=23345, PulsePeriod=0.2, PulseWidth=20, PhaseDelay=0, SwitchTimes=[0.2 0.225 0.5 0.6], LimitArcNum=off, ArcingNumber=1, AddTimeDelay=off, TimeDelay=[0 0.1 0.2 ]}
      mask prompts: FaultA "Phase A Fault"; FaultB "Phase B Fault"; FaultC "Phase C Fault"; FaultResistance "Fault resistance Ron (ohms) :"; GroundResistance "Ground resistance Rg (ohms) :"; SnubberResistance "Snubbers resistance Rp (ohms) :"; SnubberCapacitance "Snubbers capacitance Cp (F) :"; TransitionTimes "Transition times (s) :"; TheoryOfArc "Theory of the arcing ground"; ArcingVoltage "Voltage of the arcing (V) :"; TypeOfPause "Add pause in the arcing ground"; NoiseSampleTime "Sample time of white noise (s) :"; NoiseSeed "Seed of white noise"; PulsePeriod "Period of pulses (s) :"; PulseWidth "Width of pulse (% of period) :"; PhaseDelay "Phase delay (sec) :"; SwitchTimes "Switch times (sec) [1,0,1,0...] :"; LimitArcNum "Limit number of arcing [N] :"; ArcingNumber "Number of uprising arcing"; AddTimeDelay "Add time delay :"; TimeDelay "Time delay between arc (sec) [1xN] :"
      mask init: same as SPGF_FSK_0000_R2020b/K1/fault
      settings: CloseFcn=|
      | en = get_param(gcb,'MaskEnables');
      | set_param(gcb,'MaskEnables',en)
      | clear enab en;
      settings: MoveFcn=|
      | en = get_param(gcb,'MaskEnables');
      | set_param(gcb,'MaskEnables',en)
      | clear enab en;
      mask Callback FaultA:
      | enab = get_param(gcb,'FaultA');
      | en = get_param(gcb,'MaskEnables');
      | % Set the 'MaskVisililities' property for each parameters
      | if strcmp(enab,'on')
      |     en{2}='off';
      |     en{3}='off';
      | % set_param(gcb,'MaskVisibilities',{'on','on','on','on','on','on','on','on','on','off','on','',''});
      | else
      |     en{2}='on';
      |     en{3}='on';
      | % set_param(gcb,'MaskVisibilities',{'on','on','on','on','on','on','on','on','on','on','on','',''});
      | end
      | set_param(gcb,'MaskEnables',en)
      | clear enab en;
      mask Callback FaultB:
      | enab = get_param(gcb,'FaultB');
      | en = get_param(gcb,'MaskEnables');
      | % Set the 'MaskVisililities' property for each parameters
      | if strcmp(enab,'on')
      |     en{1}='off';
      |     en{3}='off';
      | % set_param(gcb,'MaskVisibilities',{'on','on','on','on','on','on','on','on','on','off','on','',''});
      | else
      |     en{1}='on';
      |     en{3}='on';
      | % set_param(gcb,'MaskVisibilities',{'on','on','on','on','on','on','on','on','on','on','on','',''});
      | end
      | set_param(gcb,'MaskEnables',en)
      | clear enab en;
      mask Callback FaultC:
      | enab = get_param(gcb,'FaultC');
      | en = get_param(gcb,'MaskEnables');
      | % Set the 'MaskVisililities' property for each parameters
      | if strcmp(enab,'on')
      |     en{1}='off';
      |     en{2}='off';
      | % set_param(gcb,'MaskVisibilities',{'on','on','on','on','on','on','on','on','on','off','on','',''});
      | else
      |     en{1}='on';
      |     en{2}='on';
      | % set_param(gcb,'MaskVisibilities',{'on','on','on','on','on','on','on','on','on','on','on','',''});
      | end
      | set_param(gcb,'MaskEnables',en)
      | clear enab en;
      mask TypeOptions TheoryOfArc: None | Petersen | Peters & Slepian
      mask Callback TheoryOfArc:
      | enab = get_param(gcb,'TheoryOfArc');
      | en = get_param(gcb,'MaskEnables');
      | % Set the 'MaskVisililities' property for each parameters
      | if strcmp(enab,'None')
      |     en{10}='off';
      | % set_param(gcb,'MaskVisibilities',{'on','on','on','on','on','on','on','on','on','off','on','',''});
      | else
      |     en{10}='on';
      | % set_param(gcb,'MaskVisibilities',{'on','on','on','on','on','on','on','on','on','on','on','',''});
      | end
      | set_param(gcb,'MaskEnables',en)
      | clear enab en;
      mask TypeOptions TypeOfPause: None | White Noise | Pulse Generator | Time Dependent Pulses
      mask Callback TypeOfPause:
      | enab = get_param(gcb,'TypeOfPause');
      | en = get_param(gcb,'MaskVisibilities');
      | % Set the 'MaskVisibilities' property for each parameters
      | if strcmp(enab,'None')
      |     en{12} = 'off';
      |     en{13} = 'off';
      |     en{14} = 'off';
      |     en{15} = 'off';
      |     en{16} = 'off';
      |     en{17} = 'off';
      | % set_param(gcb,'MaskEnables',{'on','on','on','on','on','on','on','on','on','on','on','on','on'});
      | elseif strcmp(enab,'White Noise')
      |     en{12} = 'on';
      |     en{13} = 'on';
      |     en{14} = 'off';
      |     en{15} = 'off';
      |     en{16} = 'off';
      |     en{17} = 'off';
      | elseif strcmp(enab,'Pulse Generator')
      |     en{12} = 'off';
      |     en{13} = 'off';
      |     en{14} = 'on';
      |     en{15} = 'on';
      |     en{16} = 'on';
      |     en{17} = 'off';
      | else
      |     en{12} = 'off';
      |     en{13} = 'off';
      |     en{14} = 'off';
      |     en{15} = 'off';
      |     en{16} = 'off';
      |     en{17} = 'on';
      | % set_param(gcb,'Maskenables',{'on','on','on','on','on','on','on','on','on','on','on','off','off'});
      | end
      | set_param(gcb,'MaskVisibilities',en);
      | clear enab en;
      mask Callback LimitArcNum:
      | enab = get_param(gcb,'LimitArcNum');
      | en = get_param(gcb,'MaskVisibilities');
      | % Set the 'MaskVisibilities' property for each parameters
      | if strcmp(enab,'on')
      |     en{19} = 'on';
      |     en{20} = 'on';
      |     en{21} = 'on';
      | else
      |     en{19} = 'off';
      |     en{20} = 'off';
      |     set_param(gcb,'AddTimeDelay','off');
      |     en{21} = 'off';
      | % set_param(gcb,'Maskenables',{'on','on','on','on','on','on','on','on','on','on','on','off','off'});
      | end
      | set_param(gcb,'MaskVisibilities',en);
      | clear enab en;
      mask Callback AddTimeDelay:
      | enab = get_param(gcb,'AddTimeDelay');
      | en = get_param(gcb,'MaskVisibilities');
      | % Set the 'MaskVisibilities' property for each parameters
      | if strcmp(enab,'on')
      |     en{21} = 'on';
      | else
      |     en{21} = 'off';
      | % set_param(gcb,'Maskenables',{'on','on','on','on','on','on','on','on','on','on','on','off','off'});
      | end
      | set_param(gcb,'MaskVisibilities',en);
      | clear enab en;
      mask Display:
      | % port_label('input',1,'Iabc');
      | 
      | port_label('lconn',1,'A');
      | port_label('lconn',2,'B');
      | port_label('lconn',3,'C');
      | 
      | disp('   ПДЗ    ');
  meas : Subsystem
  A : PMIOPort  Side=Left
  B : PMIOPort  Port=2  Side=Left
  C : PMIOPort  Port=3  Side=Left
  connections:
  fault/LConn1 -- meas/RConn1
  fault/LConn2 -- meas/RConn2
  fault/LConn3 -- meas/RConn3
  meas/LConn2 -- B/RConn1
  meas/LConn1 -- A/RConn1
  meas/LConn3 -- C/RConn1

== system SPGF_FSK_0000_R2020b/K3 ==
  fault : Subsystem  mask{FaultA=on, FaultB=off, FaultC=off, FaultResistance=0.0001, GroundResistance=1e-03, SnubberResistance=1e6, SnubberCapacitance=inf, TransitionTimes=[0.2 0.8], TheoryOfArc=Peters & Slepian, ArcingVoltage=[4000 9000], TypeOfPause=Time Dependent Pulses, NoiseSampleTime=0.04, NoiseSeed=23345, PulsePeriod=0.2, PulseWidth=20, PhaseDelay=0.2, SwitchTimes=[0.2 0.225 0.5 0.6], LimitArcNum=off, ArcingNumber=1, AddTimeDelay=off, TimeDelay=[0 0.1 0.2 ]}
      mask prompts: FaultA "Phase A Fault"; FaultB "Phase B Fault"; FaultC "Phase C Fault"; FaultResistance "Fault resistance Ron (ohms) :"; GroundResistance "Ground resistance Rg (ohms) :"; SnubberResistance "Snubbers resistance Rp (ohms) :"; SnubberCapacitance "Snubbers capacitance Cp (F) :"; TransitionTimes "Transition times (s) :"; TheoryOfArc "Theory of the arcing ground"; ArcingVoltage "Voltage of the arcing (V) :"; TypeOfPause "Add pause in the arcing ground"; NoiseSampleTime "Sample time of white noise (s) :"; NoiseSeed "Seed of white noise"; PulsePeriod "Period of pulses (s) :"; PulseWidth "Width of pulse (% of period) :"; PhaseDelay "Phase delay (sec) :"; SwitchTimes "Switch times (sec) [1,0,1,0...] :"; LimitArcNum "Limit number of arcing [N] :"; ArcingNumber "Number of uprising arcing"; AddTimeDelay "Add time delay :"; TimeDelay "Time delay between arc (sec) [1xN] :"
      mask init: same as SPGF_FSK_0000_R2020b/K1/fault
      settings: CloseFcn=|
      | en = get_param(gcb,'MaskEnables');
      | set_param(gcb,'MaskEnables',en)
      | clear enab en;
      settings: MoveFcn=|
      | en = get_param(gcb,'MaskEnables');
      | set_param(gcb,'MaskEnables',en)
      | clear enab en;
      mask Callback FaultA:
      | enab = get_param(gcb,'FaultA');
      | en = get_param(gcb,'MaskEnables');
      | % Set the 'MaskVisililities' property for each parameters
      | if strcmp(enab,'on')
      |     en{2}='off';
      |     en{3}='off';
      | % set_param(gcb,'MaskVisibilities',{'on','on','on','on','on','on','on','on','on','off','on','',''});
      | else
      |     en{2}='on';
      |     en{3}='on';
      | % set_param(gcb,'MaskVisibilities',{'on','on','on','on','on','on','on','on','on','on','on','',''});
      | end
      | set_param(gcb,'MaskEnables',en)
      | clear enab en;
      mask Callback FaultB:
      | enab = get_param(gcb,'FaultB');
      | en = get_param(gcb,'MaskEnables');
      | % Set the 'MaskVisililities' property for each parameters
      | if strcmp(enab,'on')
      |     en{1}='off';
      |     en{3}='off';
      | % set_param(gcb,'MaskVisibilities',{'on','on','on','on','on','on','on','on','on','off','on','',''});
      | else
      |     en{1}='on';
      |     en{3}='on';
      | % set_param(gcb,'MaskVisibilities',{'on','on','on','on','on','on','on','on','on','on','on','',''});
      | end
      | set_param(gcb,'MaskEnables',en)
      | clear enab en;
      mask Callback FaultC:
      | enab = get_param(gcb,'FaultC');
      | en = get_param(gcb,'MaskEnables');
      | % Set the 'MaskVisililities' property for each parameters
      | if strcmp(enab,'on')
      |     en{1}='off';
      |     en{2}='off';
      | % set_param(gcb,'MaskVisibilities',{'on','on','on','on','on','on','on','on','on','off','on','',''});
      | else
      |     en{1}='on';
      |     en{2}='on';
      | % set_param(gcb,'MaskVisibilities',{'on','on','on','on','on','on','on','on','on','on','on','',''});
      | end
      | set_param(gcb,'MaskEnables',en)
      | clear enab en;
      mask TypeOptions TheoryOfArc: None | Petersen | Peters & Slepian
      mask Callback TheoryOfArc:
      | enab = get_param(gcb,'TheoryOfArc');
      | en = get_param(gcb,'MaskEnables');
      | % Set the 'MaskVisililities' property for each parameters
      | if strcmp(enab,'None')
      |     en{10}='off';
      | % set_param(gcb,'MaskVisibilities',{'on','on','on','on','on','on','on','on','on','off','on','',''});
      | else
      |     en{10}='on';
      | % set_param(gcb,'MaskVisibilities',{'on','on','on','on','on','on','on','on','on','on','on','',''});
      | end
      | set_param(gcb,'MaskEnables',en)
      | clear enab en;
      mask TypeOptions TypeOfPause: None | White Noise | Pulse Generator | Time Dependent Pulses
      mask Callback TypeOfPause:
      | enab = get_param(gcb,'TypeOfPause');
      | en = get_param(gcb,'MaskVisibilities');
      | % Set the 'MaskVisibilities' property for each parameters
      | if strcmp(enab,'None')
      |     en{12} = 'off';
      |     en{13} = 'off';
      |     en{14} = 'off';
      |     en{15} = 'off';
      |     en{16} = 'off';
      |     en{17} = 'off';
      | % set_param(gcb,'MaskEnables',{'on','on','on','on','on','on','on','on','on','on','on','on','on'});
      | elseif strcmp(enab,'White Noise')
      |     en{12} = 'on';
      |     en{13} = 'on';
      |     en{14} = 'off';
      |     en{15} = 'off';
      |     en{16} = 'off';
      |     en{17} = 'off';
      | elseif strcmp(enab,'Pulse Generator')
      |     en{12} = 'off';
      |     en{13} = 'off';
      |     en{14} = 'on';
      |     en{15} = 'on';
      |     en{16} = 'on';
      |     en{17} = 'off';
      | else
      |     en{12} = 'off';
      |     en{13} = 'off';
      |     en{14} = 'off';
      |     en{15} = 'off';
      |     en{16} = 'off';
      |     en{17} = 'on';
      | % set_param(gcb,'Maskenables',{'on','on','on','on','on','on','on','on','on','on','on','off','off'});
      | end
      | set_param(gcb,'MaskVisibilities',en);
      | clear enab en;
      mask Callback LimitArcNum:
      | enab = get_param(gcb,'LimitArcNum');
      | en = get_param(gcb,'MaskVisibilities');
      | % Set the 'MaskVisibilities' property for each parameters
      | if strcmp(enab,'on')
      |     en{19} = 'on';
      |     en{20} = 'on';
      |     en{21} = 'on';
      | else
      |     en{19} = 'off';
      |     en{20} = 'off';
      |     set_param(gcb,'AddTimeDelay','off');
      |     en{21} = 'off';
      | % set_param(gcb,'Maskenables',{'on','on','on','on','on','on','on','on','on','on','on','off','off'});
      | end
      | set_param(gcb,'MaskVisibilities',en);
      | clear enab en;
      mask Callback AddTimeDelay:
      | enab = get_param(gcb,'AddTimeDelay');
      | en = get_param(gcb,'MaskVisibilities');
      | % Set the 'MaskVisibilities' property for each parameters
      | if strcmp(enab,'on')
      |     en{21} = 'on';
      | else
      |     en{21} = 'off';
      | % set_param(gcb,'Maskenables',{'on','on','on','on','on','on','on','on','on','on','on','off','off'});
      | end
      | set_param(gcb,'MaskVisibilities',en);
      | clear enab en;
      mask Display:
      | % port_label('input',1,'Iabc');
      | 
      | port_label('lconn',1,'A');
      | port_label('lconn',2,'B');
      | port_label('lconn',3,'C');
      | 
      | disp('   ПДЗ    ');
  meas : Subsystem
  A : PMIOPort  Side=Left
  B : PMIOPort  Port=2  Side=Left
  C : PMIOPort  Port=3  Side=Left
  connections:
  fault/LConn1 -- meas/RConn1
  fault/LConn2 -- meas/RConn2
  fault/LConn3 -- meas/RConn3
  meas/LConn2 -- B/RConn1
  meas/LConn1 -- A/RConn1
  meas/LConn3 -- C/RConn1
